simulink library "sunVector_lib"  (R2018b)
settings: Solver=VariableStepAuto  StartTime=0.0  StopTime=10.0  RelTol=1e-3
libraries: time_lib x1
settings Model: Creator=devantormey  LastModifiedBy=devantormey

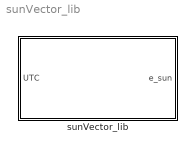
== system sunVector_lib ==
  sunVector_lib : Subsystem

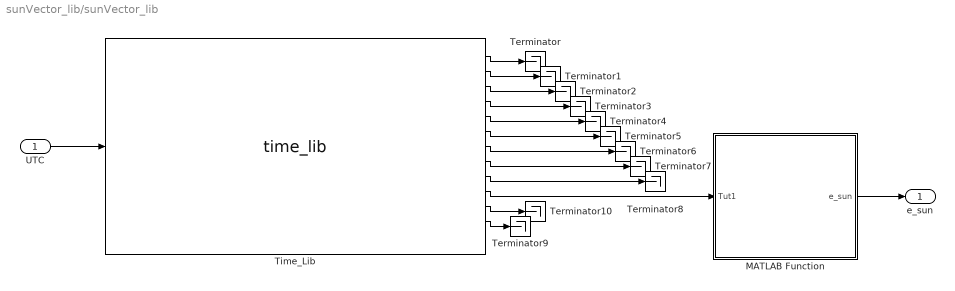
== system sunVector_lib/sunVector_lib ==
  UTC : Inport
  MATLAB Function : MATLAB Function  TreatAsAtomicUnit=on
  Terminator{,1..10} (11 alike) : Terminator
  "Time_Lib " : time_lib/time_lib    SystemSampleTime=-1
  e_sun : Outport
  wires:
  MATLAB Function/1(e_sun) -> e_sun/1
  "Time_Lib "/10 -> MATLAB Function/1(Tut1)
  "Time_Lib "/1 -> Terminator/1
  "Time_Lib "/2 -> Terminator1/1
  "Time_Lib "/3 -> Terminator2/1
  "Time_Lib "/4 -> Terminator3/1
  "Time_Lib "/5 -> Terminator4/1
  "Time_Lib "/6 -> Terminator5/1
  "Time_Lib "/7 -> Terminator6/1
  "Time_Lib "/8 -> Terminator7/1
  "Time_Lib "/9 -> Terminator8/1
  "Time_Lib "/12 -> Terminator9/1
  "Time_Lib "/11 -> Terminator10/1
  UTC/1 -> "Time_Lib "/1

== matlab function sunVector_lib/MATLAB Function ==
  data: Tut1 input; e_sun output
function e_sun = fcn(Tut1)
% DESCRIPTION
% ~~~~~~~~~~~~~
% This function computes the mean longitude phi_s and mean anomoly M_s of
% the sun from an incoming time stampe Tut1. Tut1 is computed using the
% BLANK formula
% ~~~~~~~~~~~~~~~~~~~~~~~~~~~~~~~~~~~~~~
% Variables
% Tut1 - 
% phi_s - mean longitude of sun
% M_s - mean anomoly of the sun
% phi_e - longitude of ecliptic
% eps - obliquity of the ecliptic
% e_sun - Unit vector pointing to sun
% ~~~~~~~~~~~~~~~~~~~~~~~~~~~~~~~~~~~~~~


% first compute mean longitude
phi_s = 280.460 + 36000.771*Tut1;
% Now compute mean anomoly
M_s = 357.5277233 + 35999.05034*Tut1;

% now compute longitude of the ecliptic using
phi_e = phi_s + 1.914666471*sind(M_s) + 0.019994643*sind(2*M_s);

% Obliquity of ecliptic
eps = 23.439291 - 0.0130042*Tut1;

e_sun = [cosd(phi_e);cosd(eps)*sind(phi_e); sind(eps)*sind(phi_e)];

end
